simulink model "IndustrialMicrogrid"  (R2023a)
settings: Solver=FixedStepDiscrete  StartTime=0.0  StopTime=10  FixedStep=Ts  RelTol=1e-3
PostLoadFcn:
  | IndustrialMicrogridInputData
  | GfmGridFormingConverterInputParameters
model workspace (MAT data in the model file):
  caseNum = 2
undefined symbols (not defined in the file): base, BESS, DiscIntNeverNeededParam, grid, Grid, gridInverter, machine, microgrid, PV, PVInverter, PVTransformer, scrFactorRg, scrFactorXg, transformer, Ts
libraries: ee_lib x112, eeGeneralControl x104, nesl_utility_internal x64, simulink x56, nesl_utility x37, fl_lib x29, slpidlib x13, eeTransforms x11, eeTotalHarmonicDistorsion x8, eeRmsMeasurement x4, eeSinusoidalMeasurement x4, simulink_extras x2
(part 4 of 14)

== system IndustrialMicrogrid/MG2 Processing, Lighting and Auxiliary Loads/Motor Loads ==
  ASM measurement : ee_lib/Electromechanical/Asynchronous/Induction Machine Measurement  output_idx=11
      settings: InternalSimscapePortConfiguration="{\"Bottom\":[],\"Left\":[{\"id\":\"pu_input\",\"label\":\"pu\",\"type\":\"input\"}],\"Right\":[{\"id\":\"pu_output\",\"label\":\"o\",\"type\":\"output\"}],\"Top\":[]}"
  ASM measurement1 : ee_lib/Electromechanical/Asynchronous/Induction Machine Measurement  output_idx=12
      settings: InternalSimscapePortConfiguration="{\"Bottom\":[],\"Left\":[{\"id\":\"pu_input\",\"label\":\"pu\",\"type\":\"input\"}],\"Right\":[{\"id\":\"pu_output\",\"label\":\"o\",\"type\":\"output\"}],\"Top\":[]}"
  ASM measurement2 : ee_lib/Electromechanical/Asynchronous/Induction Machine Measurement  output_idx=12
      settings: InternalSimscapePortConfiguration="{\"Bottom\":[],\"Left\":[{\"id\":\"pu_input\",\"label\":\"pu\",\"type\":\"input\"}],\"Right\":[{\"id\":\"pu_output\",\"label\":\"o\",\"type\":\"output\"}],\"Top\":[]}"
  Asynchronous Machine Squirrel Cage (fundamental) : ee_lib/Electromechanical/Asynchronous/Induction Machine Squirrel Cage  port_option=ee.enum.threePhasePort.composite  SRated=750000 V*A  VRated=4160 V  FRated=60 Hz  nPolePairs=2  param_unit=ee.enum.unit.si  squirrel_cage=ee.enum.squirrelcage.Single  zero_sequence=ee.enum.park.zerosequence.exclude  initialization_option=ee.enum.asm.initialization.steadystate  Rs=0.016744*7 Ohm  Xls=0.035490*7 Ohm  pu_Rs=0.0258  pu_Lls=0.0413  Rrd=0.009857*7 Ohm  Xlrd=0.04280*7 Ohm  pu_Rrd=0.0145  pu_Llrd=0.0424  Rrd1=0.28 Ohm  Xlrd1=0.82 Ohm  Rrd2=0.28 Ohm  Xlrd2=0.82 Ohm  pu_Rrd1=0.0290  pu_Llrd1=0.0848  pu_Rrd2=0.0290  pu_Llrd2=0.0848  Xm=111.90*7 Ohm  pu_Lm=1.7562  X0=0.4*7 Ohm  pu_L0=0.0413  saturation_option=ee.enum.saturation.exclude  saturation_i=[0, 4, 9, 18, 25, 34, 50, 68, 95, 120] A  saturation_v=[0, 88, 154, 198, 220, 242, 264, 286, 308, 327] V  pu_saturation_i=[0, .176, .396, .792, 1.1, 1.496, 2.2, 2.992, 4.18, 5.28]  pu_saturation_v=[0, .4, .7, .9, 1, 1.1, 1.2, 1.3, 1.4, 1.4864]  connection_option=ee.enum.Connection.delta1  angular_position_specify=off  angular_position_priority=None  angular_position=0 deg  angular_position_nominal_specify=off  angular_position_nominal_unit=deg  angular_position_nominal_value=1  pu_psids_specify=off  pu_psids_priority=None  pu_psids=0  pu_psids_nominal_specify=off  pu_psids_nominal_unit=1  pu_psids_nominal_value=1  pu_psiqs_specify=off  pu_psiqs_priority=None  pu_psiqs=0  pu_psiqs_nominal_specify=off  pu_psiqs_nominal_unit=1  pu_psiqs_nominal_value=1  pu_psi0s_specify=off  pu_psi0s_priority=None  pu_psi0s=0  pu_psi0s_nominal_specify=off  pu_psi0s_nominal_unit=1  pu_psi0s_nominal_value=1  pu_psidr_specify=off  pu_psidr_priority=None  pu_psidr=0  pu_psidr_nominal_specify=off  pu_psidr_nominal_unit=1  pu_psidr_nominal_value=1  pu_psiqr_specify=off  pu_psiqr_priority=None  pu_psiqr=0  pu_psiqr_nominal_specify=off  pu_psiqr_nominal_unit=1  pu_psiqr_nominal_value=1  pu_psidr1_specify=off  pu_psidr1_priority=None  pu_psidr1=0  pu_psidr1_nominal_specify=off  pu_psidr1_nominal_unit=1  pu_psidr1_nominal_value=1  pu_psiqr1_specify=off  pu_psiqr1_priority=None  pu_psiqr1=0  pu_psiqr1_nominal_specify=off  pu_psiqr1_nominal_unit=1  pu_psiqr1_nominal_value=1  pu_psidr2_specify=off  pu_psidr2_priority=None  pu_psidr2=0  pu_psidr2_nominal_specify=off  pu_psidr2_nominal_unit=1  pu_psidr2_nominal_value=1  pu_psiqr2_specify=off  pu_psiqr2_priority=None  pu_psiqr2=0  pu_psiqr2_nominal_specify=off  pu_psiqr2_nominal_unit=1  pu_psiqr2_nominal_value=1  psids_specify=off  psids_priority=None  psids=0 Wb  psids_nominal_specify=off  psids_nominal_unit=Wb  psids_nominal_value=1  psiqs_specify=off  psiqs_priority=None  psiqs=0 Wb  psiqs_nominal_specify=off  psiqs_nominal_unit=Wb  psiqs_nominal_value=1  psi0s_specify=off  psi0s_priority=None  psi0s=0 Wb  psi0s_nominal_specify=off  psi0s_nominal_unit=Wb  psi0s_nominal_value=1  psidr_specify=off  psidr_priority=None  psidr=0 Wb  psidr_nominal_specify=off  psidr_nominal_unit=Wb  psidr_nominal_value=1  psiqr_specify=off  psiqr_priority=None  psiqr=0 Wb  psiqr_nominal_specify=off  psiqr_nominal_unit=Wb  psiqr_nominal_value=1  psidr1_specify=off  psidr1_priority=None  psidr1=0 Wb  psidr1_nominal_specify=off  psidr1_nominal_unit=Wb  psidr1_nominal_value=1  psiqr1_specify=off  psiqr1_priority=None  psiqr1=0 Wb  psiqr1_nominal_specify=off  psiqr1_nominal_unit=Wb  psiqr1_nominal_value=1  psidr2_specify=off  psidr2_priority=None  psidr2=0 Wb  psidr2_nominal_specify=off  psidr2_nominal_unit=Wb  psidr2_nominal_value=1  psiqr2_specify=off  psiqr2_priority=None  psiqr2=0 Wb  psiqr2_nominal_specify=off  psiqr2_nominal_unit=Wb  psiqr2_nominal_value=1  slip_specify=off  slip_priority=None  slip=0  slip_nominal_specify=off  slip_nominal_unit=1  slip_nominal_value=1  real_power_generated_specify=off  real_power_generated_priority=None  real_power_generated=0 W  real_power_generated_nominal_specify=off  real_power_generated_nominal_unit=W  real_power_generated_nominal_value=1  mechanical_power_consumed_specify=off  mechanical_power_consumed_priority=None  mechanical_power_consumed=0 W  mechanical_power_consumed_nominal_specify=off  mechanical_power_consumed_nominal_unit=W  mechanical_power_consumed_nominal_value=1  Tmeas=298.15 K  alpha=3.93e-3 1/K  alpha_cage=4.4e-3 1/K  stator_thermal_mass=100 J/K  rotor_thermal_mass=200 J/K  temperatureA_specify=off  temperatureA_priority=High  temperatureA=25 degC  temperatureA_nominal_specify=off  temperatureA_nominal_unit=degC  temperatureA_nominal_value=1  temperatureB_specify=off  temperatureB_priority=High  temperatureB=25 degC  temperatureB_nominal_specify=off  temperatureB_nominal_unit=degC  temperatureB_nominal_value=1  temperatureC_specify=off  temperatureC_priority=High  temperatureC=25 degC  temperatureC_nominal_specify=off  temperatureC_nominal_unit=degC  temperatureC_nominal_value=1  temperatureR_specify=off  temperatureR_priority=High  temperatureR=25 degC  temperatureR_nominal_specify=off  temperatureR_nominal_unit=degC  temperatureR_nominal_value=1
      settings: InternalSimscapePortConfiguration="{\"Bottom\":[],\"Left\":[{\"id\":\"R\",\"label\":\"R\",\"type\":\"foundation.mechanical.rotational.rotational\"},{\"id\":\"C\",\"label\":\"C\",\"type\":\"foundation.mechanical.rotational.rotational\"}],\"Right\":[{\"id\":\"pu_output\",\"label\":\"pu\",\"type\":\"output\"},{\"id\":\"N1\",\"label\":\"~1\",\"type\":\"foundation.electrical.three_phase\"},{\"id\":\"N2\",\"label\":\"~2\",\"type\":\"foundation.electrical.three_phase\"}],\"Top\":[]}"
  Electrical Reference1 : fl_lib/Electrical/Electrical Elements/Electrical Reference
  Generator : Scope  NumInputPorts=3
  Generator Sign Convention : Gain  Gain=-1
  Generator Sign Convention1 : Gain  Gain=-1
  Neutral Port (Three-Phase) : ee_lib/Connectors & References/Neutral Port (Three-Phase)  G_parasitic=1e-12 1/Ohm
      settings: InternalSimscapePortConfiguration="{\"Bottom\":[],\"Left\":[{\"id\":\"N\",\"label\":\"~\",\"type\":\"foundation.electrical.three_phase\"}],\"Right\":[{\"id\":\"n\",\"label\":\"n\",\"type\":\"foundation.electrical.electrical\"}],\"Top\":[]}"
  PS-Simulink Converter1 : nesl_utility/PS-Simulink Converter  PhysicalDomain=network_engine_domain  SubClassName=ps_output  LeftPortType=input  RightPortType=output  PseudoPeriodic=off  Frequencies=[]  VectorFormat=1-D array  Unit=1  AffineConversion=off
  PS-Simulink Converter2 : nesl_utility/PS-Simulink Converter  PhysicalDomain=network_engine_domain  SubClassName=ps_output  LeftPortType=input  RightPortType=output  PseudoPeriodic=off  Frequencies=[]  VectorFormat=1-D array  Unit=1  AffineConversion=off
  PS-Simulink Converter3 : nesl_utility/PS-Simulink Converter  PhysicalDomain=network_engine_domain  SubClassName=ps_output  LeftPortType=input  RightPortType=output  PseudoPeriodic=off  Frequencies=[]  VectorFormat=1-D array  Unit=1  AffineConversion=off
  Subsystem : Subsystem
  Two-Winding Transformer (Three-Phase)1 : ee_lib/Passive/Transformers/Two-Winding Transformer (Three-Phase)  SRated=microgrid.unitSubstationTransformerRating A*V  FRated=microgrid.frequency Hz  Winding1Connection=ee.enum.windingconnection.Y  VRated1=microgrid.powerCenterVoltage V  Winding2Connection=ee.enum.windingconnection.Y  VRated2=microgrid.powerCenterVoltage V  CoreType=ee.enum.coretype.threelimb  pu_Rw1=microgrid.unitSubstationPrimaryResistance  pu_Rw2=microgrid.unitSubstationPrimaryReactance*2  leakage_reactance_option=ee.enum.transformer_leakage.include  pu_Xl1=microgrid.unitSubstationSecondaryResistance  pu_Xl2=microgrid.unitSubstationSecondaryReactance*2  magnetizing_resistance_option=ee.enum.transformer_magnetizingResistance.include  pu_Rm=500  magnetizing_reactance_option=ee.enum.transformer_magnetizingReactance.include  saturation_option=ee.enum.transformer_saturation.exclude  pu_Xm=500  current_data=[0, .002, 1, 2]  magnetic_flux_data=[0, 1.2, 1.5, 1.51]  pu_X0=0.5  i1_specify=on  i1_priority=None  i1=[0, 0, 0] A  i1_nominal_specify=off  i1_nominal_unit=A  i1_nominal_value=1  i2_specify=on  i2_priority=None  i2=[0, 0, 0] A  i2_nominal_specify=off  i2_nominal_unit=A  i2_nominal_value=1  phi_specify=off  phi_priority=None  phi=[0, 0, 0]  phi_nominal_specify=off  phi_nominal_unit=1  phi_nominal_value=1  power_dissipated_specify=off  power_dissipated_priority=None  power_dissipated=0 W  power_dissipated_nominal_specify=off  power_dissipated_nominal_unit=W  power_dissipated_nominal_value=1
      settings: InternalSimscapePortConfiguration="{\"Bottom\":[],\"Left\":[{\"id\":\"N1\",\"label\":\"~1\",\"type\":\"foundation.electrical.three_phase\"}],\"Right\":[{\"id\":\"N2\",\"label\":\"~2\",\"type\":\"foundation.electrical.three_phase\"}],\"Top\":[]}"
  Conn2 : PMIOPort  Side=Right
  wires:
  PS-Simulink Converter1/1 -> Generator Sign Convention1/1
  Generator Sign Convention/1 -> Generator/1  "Real Power, pu"
  PS-Simulink Converter2/1 -> Generator Sign Convention/1
  Generator Sign Convention1/1 -> Generator/2  "Reactive Power, pu"
  PS-Simulink Converter3/1 -> Generator/3
  connections:
  ASM measurement/LConn1 -- ASM measurement1/LConn1 -- Asynchronous Machine Squirrel Cage (fundamental)/RConn1 -- ASM measurement2/LConn1
  Subsystem/LConn2 -- Asynchronous Machine Squirrel Cage (fundamental)/LConn2
  Subsystem/LConn1 -- Asynchronous Machine Squirrel Cage (fundamental)/LConn1
  Neutral Port (Three-Phase)/RConn1 -- Electrical Reference1/LConn1
  ASM measurement/RConn1 -- PS-Simulink Converter2/LConn1
  Two-Winding Transformer (Three-Phase)1/RConn1 -- Conn2/RConn1
  Asynchronous Machine Squirrel Cage (fundamental)/RConn3 -- Neutral Port (Three-Phase)/LConn1
  PS-Simulink Converter3/LConn1 -- ASM measurement2/RConn1
  ASM measurement1/RConn1 -- PS-Simulink Converter1/LConn1
  Asynchronous Machine Squirrel Cage (fundamental)/RConn2 -- Two-Winding Transformer (Three-Phase)1/LConn1

== system IndustrialMicrogrid/Operator Room/OperatorControlRoom ==
  mLoad : Inport
  mLoad2 : Inport  Port=2
  MGController2 : Inport  Port=3
  mPV : Inport  Port=4
  MGController1 : Inport  Port=5
  Tieline1 : Inport  Port=6
  mLoad3 : Inport  Port=7
  mDiesel : Inport  Port=8
  Tieline : Inport  Port=9
  "MG1 Controller : Commands and Measurements" : Subsystem
  "MG2 Controller : Commands and Measurements" : Subsystem
  Control Room MG1 : Outport
  Control Room MG2 : Outport  Port=2
  wires:
  mLoad/1 -> "MG1 Controller : Commands and Measurements"/1(mLoad)
  MGController1/1 -> "MG1 Controller : Commands and Measurements"/2(MGController1)
  "MG1 Controller : Commands and Measurements"/1(ControlRoom) -> Control Room MG1/1
  mLoad2/1 -> "MG2 Controller : Commands and Measurements"/1(mLoad2)
  MGController2/1 -> "MG2 Controller : Commands and Measurements"/2(MGController2)
  mPV/1 -> "MG2 Controller : Commands and Measurements"/3(mPV)
  mDiesel/1 -> "MG2 Controller : Commands and Measurements"/4(mDiesel)
  "MG2 Controller : Commands and Measurements"/1(ControlRoom) -> Control Room MG2/1
  Tieline1/1 -> "MG1 Controller : Commands and Measurements"/3(Tieline)
  Tieline/1 -> "MG2 Controller : Commands and Measurements"/5(mTieline)
  mLoad3/1 -> "MG1 Controller : Commands and Measurements"/4(mLoad3)

== system IndustrialMicrogrid/Operator Room/Signal Selector ==
  Control Room MG1 : Inport
  Control Room MG2 : Inport  Port=2
  "Control Room MG1 " : InportShadow
  Control Room MG1 1 : InportShadow
  Control Room MG1 2 : InportShadow
  "Control Room MG2 " : InportShadow  Port=2
  Control Room MG2 1 : InportShadow  Port=2
  MG1 Load : Subsystem
  MG1 Portable Substation : Subsystem
  MG1 Primary Substation : Subsystem
  MG1 Unit Substation : Subsystem
  MG2 Load : Subsystem
  MG2 Power Center : Subsystem
  MG2 Primary Substation : Subsystem
  Primary Substation 1 : Outport
  Primary Substation 2 : Outport  Port=2
  Unit Substation : Outport  Port=3
  Power Center : Outport  Port=4
  Drilling Load : Outport  Port=5
  "Processing, and Auxiliary Loads " : Outport  Port=6
  Portable Substation : Outport  Port=7
  wires:
  Control Room MG1/1 -> MG1 Primary Substation/1(In1)
  MG1 Primary Substation/1(Primary Substation 1) -> Primary Substation 1/1
  Control Room MG2/1 -> MG2 Primary Substation/1(In1)
  MG2 Primary Substation/1(Primary Substation 2) -> Primary Substation 2/1
  "Control Room MG1 "/1 -> MG1 Unit Substation/1(In1)
  MG1 Unit Substation/1(Out1) -> Unit Substation/1
  "Control Room MG2 "/1 -> MG2 Power Center/1(In1)
  MG2 Power Center/1(Out1) -> Power Center/1
  Control Room MG1 1/1 -> MG1 Load/1(In1)
  MG1 Load/1(Out1) -> Drilling Load/1
  Control Room MG2 1/1 -> MG2 Load/1(In1)
  MG2 Load/1(Out1) -> "Processing, and Auxiliary Loads "/1
  Control Room MG1 2/1 -> MG1 Portable Substation/1(In1)
  MG1 Portable Substation/1(Portable Substation) -> Portable Substation/1

== system IndustrialMicrogrid/Selected Results/MG1 ==
  In Bus Element29 : Inport  PortName=MGController1  Element=BESS.active power
  In Bus Element30 : Inport  PortName=MGController1  Element=BESS.reactive power
  In Bus Element1 : Inport  PortName=MGController1  Element=BESS.voltage
  In Bus Element3 : Inport  PortName=MGController1  Element=BESS.voltage
  In Bus Element2 : Inport  PortName=MGController1  Element=BESS.current
  In Bus Element4 : Inport  PortName=MGController1  Element=BESS.current
  In Bus Element27 : Inport  PortName=MGController1  Element=Controller.ResynchMGController.PCC measurments.PCC.mPCC.activepower
  In Bus Element28 : Inport  PortName=MGController1  Element=Controller.ResynchMGController.PCC measurments.PCC.mPCC.reactivepower
  In Bus Element25 : Inport  Port=2  PortName=mLoad  Element=active power
  In Bus Element26 : Inport  Port=2  PortName=mLoad  Element=reactive power
  BESS Measurements : Scope  NumInputPorts=4
  Bus Creator : BusCreator  Inputs=3
  Bus Creator1 : BusCreator  Inputs=3
  Gain : Gain
  Gain1 : Gain
  "Inverter Active & Reactive Power " : Subsystem
  Power  Measurements : Scope  NumInputPorts=2
  Terminator : Terminator
  Terminator1 : Terminator
  wires:
  In Bus Element29/1 -> Bus Creator/2  "BESS Active Power"
  Bus Creator/1 -> Power  Measurements/1
  In Bus Element30/1 -> Bus Creator1/2  "BESS Reactive Power"
  Bus Creator1/1 -> Power  Measurements/2
  In Bus Element25/1 -> Bus Creator/3  "Load Active Power"
  In Bus Element27/1 -> Bus Creator/1  "Grid Active Power"
  In Bus Element28/1 -> Bus Creator1/1  "Grid Reactive Power"
  In Bus Element26/1 -> Bus Creator1/3  "Load Reactive Power"
  In Bus Element4/1 -> BESS Measurements/4  "BESS Current (pu)"
  "Inverter Active & Reactive Power "/2(Q) -> Gain1/1, BESS Measurements/2  "BESS  Reactive Power (pu)"
  In Bus Element2/1 -> "Inverter Active & Reactive Power "/2(Iabc)  "BESS Current (pu)"
  In Bus Element3/1 -> BESS Measurements/3  "BESS Voltage (pu)"
  "Inverter Active & Reactive Power "/1(P) -> Gain/1, BESS Measurements/1  "BESS  Active Power (pu)"
  In Bus Element1/1 -> "Inverter Active & Reactive Power "/1(Vabc)  "BESS Voltage (pu)"
  Gain/1 -> Terminator/1  "P BESS MG1"
  Gain1/1 -> Terminator1/1  "Q BESS MG1"

== system IndustrialMicrogrid/Selected Results/MG2 ==
  In Bus Element12 : Inport  PortName=MGController2  Element=BESS2.active power
  In Bus Element13 : Inport  PortName=MGController2  Element=BESS2.reactive power
  In Bus Element5 : Inport  PortName=MGController2  Element=BESS2.voltage
  In Bus Element7 : Inport  PortName=MGController2  Element=BESS2.voltage
  In Bus Element6 : Inport  PortName=MGController2  Element=BESS2.current
  In Bus Element8 : Inport  PortName=MGController2  Element=BESS2.current
  In Bus Element10 : Inport  PortName=MGController2  Element=MGController2.IslandMGController2.PCC measurments2.PCC2.mPCC2.activepower
  In Bus Element11 : Inport  PortName=MGController2  Element=MGController2.ResynchMGController2.PCC measurments2.PCC2.mPCC2.reactivepower
  In Bus Element14 : Inport  Port=2  PortName=mLoad2  Element=active power
  In Bus Element15 : Inport  Port=2  PortName=mLoad2  Element=reactive power
  In Bus Element17 : Inport  Port=3  PortName=mPV  Element=mPV.ActivePower
  In Bus Element18 : Inport  Port=3  PortName=mPV  Element=mPV.RectivePower
  In Bus Element19 : Inport  Port=4  PortName=mdiesel  Element=active power
  In Bus Element20 : Inport  Port=4  PortName=mdiesel  Element=reactive power
  BESS Measurements1 : Scope  NumInputPorts=4
  Bus Creator2 : BusCreator  Commented=on  Inputs=5
  Bus Creator3 : BusCreator  Commented=on  Inputs=5
  Bus Creator4 : BusCreator  Inputs=5
  Bus Creator5 : BusCreator  Inputs=5
  Gain : Gain
  Gain1 : Gain
  Inverter Active & Reactive Power 1 : Subsystem
  Power  Measurements1 : Scope  NumInputPorts=2
  Terminator : Terminator
  Terminator1 : Terminator
  wires:
  In Bus Element8/1 -> BESS Measurements1/4  "BESS Current (pu)"
  In Bus Element7/1 -> BESS Measurements1/3  "BESS Voltage (pu)"
  In Bus Element6/1 -> Inverter Active & Reactive Power 1/2(Iabc)  "BESS Active Power"
  In Bus Element5/1 -> Inverter Active & Reactive Power 1/1(Vabc)  "BESS Active Power"
  Bus Creator5/1 -> Power  Measurements1/2
  In Bus Element15/1 -> Bus Creator5/3  "Load Reactive Power"
  In Bus Element12/1 -> Bus Creator4/2  "BESS Active Power"
  In Bus Element17/1 -> Bus Creator4/4  "PV Active Power"
  In Bus Element10/1 -> Bus Creator4/1  "Grid Active Power"
  In Bus Element20/1 -> Bus Creator5/5  "Diesel Reactive Power"
  In Bus Element13/1 -> Bus Creator5/2  "BESS Reactive Power"
  In Bus Element11/1 -> Bus Creator5/1  "Grid Reactive Power"
  In Bus Element19/1 -> Bus Creator4/5  "Diesl Active Power"
  In Bus Element18/1 -> Bus Creator5/4  "PV Rective Power"
  In Bus Element14/1 -> Bus Creator4/3  "Load Active Power"
  Bus Creator4/1 -> Power  Measurements1/1
  Gain1/1 -> Terminator1/1  "Q BESS MG2"
  Gain/1 -> Terminator/1  "P BESS MG2"
  Inverter Active & Reactive Power 1/1(P) -> Gain/1, BESS Measurements1/1  "BESS  Active Power (pu)"
  Inverter Active & Reactive Power 1/2(Q) -> Gain1/1, BESS Measurements1/2  "BESS  Reactive Power (pu)"

== system IndustrialMicrogrid/MG1 Drilling Loads/Subsystem2/Subsystem ==
  Gain : Gain  Gain=60/(2*pi)
  Ideal Rotational Motion Sensor : fl_lib/Mechanical/Mechanical Sensors/Ideal Rotational Motion Sensor  reference=foundation.enum.MeasurementReference.difference  acceleration_port=false  velocity_port=true  position_port=false  wrap_angle=false  offset=0 rad
      settings: InternalSimscapePortConfiguration="{\"Bottom\":[],\"Left\":[{\"id\":\"R\",\"label\":\"R\",\"type\":\"foundation.mechanical.rotational.rotational\"}],\"Right\":[{\"id\":\"C\",\"label\":\"C\",\"type\":\"foundation.mechanical.rotational.rotational\"},{\"id\":\"W\",\"label\":\"W\",\"type\":\"output\"}],\"Top\":[]}"
  Machine Mechanical Power : ee_lib/Electromechanical/Mechanical/Machine Mechanical Power  power_sign=1  SRated=132000 A*V  FRated=60 Hz  nPolePairs=2  inputUnit=ee.enum.unit.si  torque_factor=2  inertia_option=2  J=10 kg*m^2  H=3.525 W*s/(A*V)  damper_option=2  D=39.0509 N*m*s/rad  pu_D=0.01  initialization_option=2  fMechanical0=60 Hz  fElectrical0=60 Hz
      settings: InternalSimscapePortConfiguration="{\"Bottom\":[],\"Left\":[{\"id\":\"Pm\",\"label\":\"Pm\",\"type\":\"input\"}],\"Right\":[{\"id\":\"R\",\"label\":\"R\",\"type\":\"foundation.mechanical.rotational.rotational\"},{\"id\":\"C\",\"label\":\"C\",\"type\":\"foundation.mechanical.rotational.rotational\"}],\"Top\":[]}"
  Mechanical Rotational Reference : fl_lib/Mechanical/Rotational Elements/Mechanical Rotational Reference
  PS-Simulink Converter : nesl_utility/PS-Simulink Converter  PhysicalDomain=network_engine_domain  SubClassName=ps_output  LeftPortType=input  RightPortType=output  PseudoPeriodic=off  Frequencies=[]  VectorFormat=inherit  Unit=inherit  AffineConversion=off
  Power : Constant  Value=120000
  Scope : Scope
  Simulink-PS Converter2 : nesl_utility/Simulink-PS Converter  PhysicalDomain=network_engine_domain  SubClassName=ps_input  LeftPortType=input  RightPortType=output  PseudoPeriodic=off  Frequencies=[]  NoiseDistribution=none  NoiseParameters=[]  Unit=1  AffineConversion=off  FilteringAndDerivatives=provide  SimscapeFilterOrder=1  InputFilterTimeConstant=0.001  UdotUserProvided=0
  Conn1 : PMIOPort  Side=Left
  Conn2 : PMIOPort  Port=2  Side=Left
  wires:
  PS-Simulink Converter/1 -> Gain/1
  Gain/1 -> Scope/1
  Power/1 -> Simulink-PS Converter2/1
  connections:
  PS-Simulink Converter/LConn1 -- Ideal Rotational Motion Sensor/RConn2
  Simulink-PS Converter2/RConn1 -- Machine Mechanical Power/LConn1
  Conn1/RConn1 -- Ideal Rotational Motion Sensor/LConn1 -- Machine Mechanical Power/RConn1
  Conn2/RConn1 -- Mechanical Rotational Reference/LConn1 -- Machine Mechanical Power/RConn2 -- Ideal Rotational Motion Sensor/RConn1

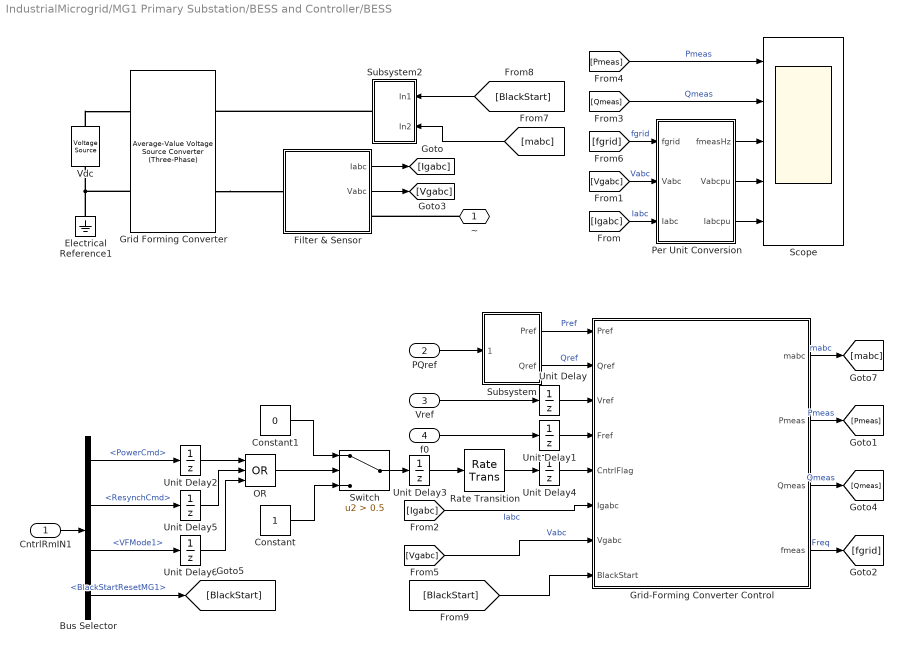
== system IndustrialMicrogrid/MG1 Primary Substation/BESS and Controller/BESS ==
  CntrlRmIN1 : Inport
  PQref : Inport  Port=2
  Vref : Inport  Port=3
  f0 : Inport  Port=4
  Bus Selector : BusSelector  OutputSignals=PowerCmd,ResynchCmd,VFMode1,BlackStartResetMG1
  Constant : Constant
  Constant1 : Constant  Value=0
  Electrical Reference1 : fl_lib/Electrical/Electrical Elements/Electrical Reference
  Filter & Sensor : Subsystem
      mask Display: image('$imagefile'); % Use "Edit Image" on toolstrip to change.
  Grid Forming Converter : ee_lib/Semiconductors & Converters/Converters/Average-Value Voltage Source Converter (Three-Phase)  port_option=ee.enum.threePhasePort.composite  frequency_option=ee.enum.converters.frequency.variable  FRated=50 Hz  losses_parameterization=ee.enum.converters.losses.fixed  Pfixed=1 W  ks=0.01  kc1=1.7 V  kc2=0.01 Ohm  Ploss_vect=[100, 800, 1870, 3250, 4900] W  Irms_vect=[10, 100, 200, 300, 400] A  Vdc_nom=300 V  thermal_mass=30000 J/K  temperature_specify=off  temperature_priority=High  temperature=298.15 K  temperature_nominal_specify=off  temperature_nominal_unit=K  temperature_nominal_value=1
      settings: InternalSimscapePortConfiguration="{\"Bottom\":[],\"Left\":[{\"id\":\"ModWave\",\"label\":\"ModWave\",\"type\":\"input\"},{\"id\":\"N\",\"label\":\"~\",\"type\":\"foundation.electrical.three_phase\"}],\"Right\":[{\"id\":\"p\",\"label\":\"+\",\"type\":\"foundation.electrical.electrical\"},{\"id\":\"n\",\"label\":\"-\",\"type\":\"foundation.electrical.electrical\"}],\"Top\":[]}"
  Grid-Forming Converter Control : Subsystem  mask(Grid Forming Controller){power=gridInverter.apparentPower*1e3, girdLineVoltage=gridInverter.lineRMSVoltage, powerFreq=gridInverter.frequency, dcBusVoltage=gridInverter.DCVoltage, measSampleTime=gridInverter.measurementSampleTime, powerControl=Virtual Synchronous Machine, activePowerSampleTime=gridInverter.droopControl.sampleTime, droopSlope=gridInverter.droopControl.freqSlopeMp, droopT1=gridInverter.droopControl.T1, droopT2=gridInverter.droopControl.T2, droopTC=gridInverter.droopControl.lpfTimeConst, vsmPmeasFilterTC=gridInverter.vsm.PmeasTimeConst, vsmFreqDroop=gridInverter.vsm.freqDroop, vsmInertiaTC=gridInverter.vsm.inertiaConstant, vsmDampingConst=gridInverter.vsm.dampingCoefficent, dampingPowerMaxLimit=gridInverter.vsm.maxDampingPower, dampingPowerMinLimit=gridInverter.vsm.minDampingPower, freqMeasTimeConst=gridInverter.freqMeasTimeConst, freqOption=Constant Frequency Reference, voltreference=gridInverter.Qcontrol.voltageReference, QVoltFilterTC=gridInverter.Qcontrol.QmeasTimeConst, QVoltDroop=gridInverter.Qcontrol.voltageDroop, currentLimit=Virtual Impedance, maxSatCurrentLimit=gridInverter.currentLimit.maxSaturationCurrent, maxVICurrentLimit=gridInverter.currentLimit.viCurrentLimit, ctLimitVirtualImp=gridInverter.currentLimit.virImpResistanceCoeff, ctLimitXbyR=gridInverter.currentLimit.virImpXbyR, ctLimitDelayTime=gridInverter.currentLimit.maxSaturationDelay, currentSatTime=gridInverter.currentLimit.satCurrentRunTime, currentVITimeConst=gridInverter.currentLimit.viFilterTimeConst, voltControlTs=gridInverter.controller.VoltageControlSampleTime, vdPGain=gridInverter.controller.voltControllerKp, VdIGain=gridInverter.controller.voltControllerKi, VdMaxCt=gridInverter.controller.voltageMaxId, VdMinCt=gridInverter.controller.voltageMinId, VqPGain=gridInverter.controller.voltControllerKp, VqIGain=gridInverter.controller.voltControllerKi, VqMaxCt=gridInverter.controller.voltageMaxIq, VqMinCt=gridInverter.controller.voltageMinIq, vdvqLPFTimeConst=gridInverter.controller.voltMeasTimeConst, currentControlTs=gridInverter.controller.CurrentControlSampleTime, filterInductance=gridInverter.L, IdPGain=gridInverter.controller.ctControllerKp, IdIGain=gridInverter.controller.ctControllerKi, IqPGain=gridInverter.controller.ctControllerKp, IqIGain=gridInverter.controller.ctControllerKi}
      mask prompts: power "Grid forming converter power (VA)"; girdLineVoltage "Grid line voltage (V)"; powerFreq "Grid frequency (Hz)"; dcBusVoltage "DC bus voltage"; measSampleTime "Measurement sample time"; powerControl "Active Power Control"; activePowerSampleTime "Sample time (s)"; droopSlope "Power droop slope (pu, Hz/W)"; droopT1 "Lead-Lag numerator time constant (s)"; droopT2 "Lead-Lag denominator time constant (s)"; droopTC "Filter cut-off time constant (s)"; vsmPmeasFilterTC "Power measurement filter time constant (s)"; vsmFreqDroop "Frequency droop (pu,  W/Hz)"; vsmInertiaTC "Inertia constant M (pu)"; vsmDampingConst "Damping constant (pu/Hz)"; dampingPowerMaxLimit "Damping power maximum limit (pu)"; dampingPowerMinLimit "Damping power minimum limit (pu)"; freqMeasTimeConst "Frequency measurement time constant (s)"; freqOption "Damping power fequency option"; voltreference "Voltage reference value (pu)"; QVoltFilterTC "Power measurement filter time constant (s)"; QVoltDroop "Voltage droop (pu, V/VAR)"; currentLimit "Current limiting method"; maxSatCurrentLimit "Maximum current saturation (pu)"; maxVICurrentLimit "Maximum virtual impedance current (pu)"; ctLimitVirtualImp "Virtual impedance coefficient (pu.Ohm/pu.A)"; ctLimitXbyR "Virtual X/R ratio"; ctLimitDelayTime "Maximum current delay time (s)"; currentSatTime "Current limiting run time (s)"; currentVITimeConst "Filter time constant (s)"; voltControlTs "Controller sample time (s)"; vdPGain "Vd proportional gain"; VdIGain "Vd integral gain"; VdMaxCt "Vd maximum current limit (A)"; VdMinCt "Vd minimum current limit (A)"; VqPGain "Vq proportional gain"; VqIGain "Vq integral gain"; VqMaxCt "Vq maximum current limit (A)"; VqMinCt "Vq minimum current limit (A)"; vdvqLPFTimeConst "Voltage measurement filter time constant (s)"; currentControlTs "Controller sample time (s)"; filterInductance "Filter inductance (H)"; IdPGain "Id proportional gain"; IdIGain "Id integral gain"; IqPGain "Iq proportional gain"; IqIGain "Iq integral gain"
      mask help: This block implements the grid forming controller with fault ride through capability. Input to the controller are active and reactive power reference in per unit and the sensed three-phase phase current in amphere and phase voltage in volts.
      mask init:
      | powerChoice = get_param(gcb,'powerControl');
      | currentChoice = get_param(gcb,'currentLimit');
      | 
      | powerloc = [gcb, '/Power Control/ActivePowerControl']; 
      | currentloc = [gcb, '/Current Limiting/CurrentLimitingMethod'];
      | freqLoc = [gcb,'/Power Control/ActivePowerControl/vsmControl/Damping Frequency'];
      | 
      | switch powerChoice
      |     case 'Virtual Synchronous Machine'
      |         set_param(powerloc, 'LabelModeActiveChoice', 'vsm');
      |         dampingFreqChoice = get_param(gcb,'freqOption');
      |         if strcmp(dampingFreqChoice,'Use Grid Frequency Measurement')
      |             set_param(freqLoc, 'LabelModeActiveChoice', 'freqMeas');
      |         else
      |             set_param(freqLoc, 'LabelModeActiveChoice', 'constFreq');
      |         end
      |     case 'Droop Control'
      |          set_param(powerloc, 'LabelModeActiveChoice', 'droop');
      |    otherwise
      |         disp('Choose proper active power control method')
      | end
      | switch currentChoice
      |     case 'Virtual Impedance'
      |           set_param(currentloc, 'LabelModeActiveChoice', 'virimp');
      |     case 'Current Limiting'
      |          set_param(currentloc, 'LabelModeActiveChoice', 'ctSat');
      |     case 'Combining Virtual Impedance and Current Limiting'
      |             set_param(currentloc, 'LabelModeActiveChoice', 'both');
      |     otherwise
      |         disp('Choose proper current limiting method')
      | end
      mask TypeOptions powerControl: Virtual Synchronous Machine | Droop Control
      mask Callback powerControl:
      | h = Simulink.Mask.get(gcb);
      | slectedActivePowerControl=get_param(gcb,'powerControl');
      | %slectedActivePowerControl = h.Parameters(find(string({h.Parameters.Name}) == 'powerControl')).Value;
      | switch slectedActivePowerControl
      |     case 'Virtual Synchronous Machine'
      |         h.Parameters(find(string({h.Parameters.Name}) == 'droopSlope')).Visible = 'off';
      |         h.Parameters(find(string({h.Parameters.Name}) == 'droopTC')).Visible = 'off';
      |         h.Parameters(find(string({h.Parameters.Name}) == 'droopT1')).Visible = 'off';
      |         h.Parameters(find(string({h.Parameters.Name}) == 'droopT2')).Visible = 'off';
      |         h.Parameters(find(string({h.Parameters.Name}) == 'vsmPmeasFilterTC')).Visible = 'on';
      |         h.Parameters(find(string({h.Parameters.Name}) == 'vsmFreqDroop')).Visible = 'on';
      |         h.Parameters(find(string({h.Parameters.Name}) == 'vsmInertiaTC')).Visible = 'on';
      |         h.Parameters(find(string({h.Parameters.Name}) == 'vsmDampingConst')).Visible = 'on';
      |         h.Parameters(find(string({h.Parameters.Name}) == 'dampingPowerMaxLimit')).Visible = 'on';
      |         h.Parameters(find(string({h.Parameters.Name}) == 'dampingPowerMinLimit')).Visible = 'on';
      |         h.Parameters(find(string({h.Parameters.Name}) == 'freqOption')).Visible = 'on';
      |         h.Parameters(find(string({h.Parameters.Name}) == 'freqMeasTimeConst')).Visible = 'on';
      |     case 'Droop Control'
      |         h.Parameters(find(string({h.Parameters.Name}) == 'droopSlope')).Visible = 'on';
      |         h.Parameters(find(string({h.Parameters.Name}) == 'droopTC')).Visible = 'on';
      |         h.Parameters(find(string({h.Parameters.Name}) == 'droopT1')).Visible = 'on';
      |         h.Parameters(find(string({h.Parameters.Name}) == 'droopT2')).Visible = 'on';
      |         h.Parameters(find(string({h.Parameters.Name}) == 'vsmPmeasFilterTC')).Visible = 'off';
      |         h.Parameters(find(string({h.Parameters.Name}) == 'vsmFreqDroop')).Visible = 'off';
      |         h.Parameters(find(string({h.Parameters.Name}) == 'vsmInertiaTC')).Visible = 'off';
      |         h.Parameters(find(string({h.Parameters.Name}) == 'vsmDampingConst')).Visible = 'off';
      |         h.Parameters(find(string({h.Parameters.Name}) == 'dampingPowerMaxLimit')).Visible = 'off';
      |         h.Parameters(find(string({h.Parameters.Name}) == 'dampingPowerMinLimit')).Visible = 'off';
      |         h.Parameters(find(string({h.Parameters.Name}) == 'freqOption')).Visible = 'off';
      |         h.Parameters(find(string({h.Parameters.Name}) == 'freqMeasTimeConst')).Visible = 'on';
      | 
      |     otherwise
      |         disp('Choose proper active power control method')
      | end
      mask TypeOptions freqOption: Use Grid Frequency Measurement | Constant Frequency Reference
      mask TypeOptions currentLimit: Virtual Impedance | Current Limiting | Combining Virtual Impedance and Current Limiting
      mask Callback currentLimit:
      | currentLimit = 1;
      | h = Simulink.Mask.get(gcb);
      | currentLimitControl=get_param(gcb,'currentLimit');
      | %slectedActivePowerControl = h.Parameters(find(string({h.Parameters.Name}) == 'powerControl')).Value;
      | switch currentLimitControl
      |     case 'Virtual Impedance'
      |         h.Parameters(find(string({h.Parameters.Name}) == 'maxVICurrentLimit')).Visible = 'on';
      |         h.Parameters(find(string({h.Parameters.Name}) == 'ctLimitVirtualImp')).Visible = 'on';
      |         h.Parameters(find(string({h.Parameters.Name}) == 'ctLimitXbyR')).Visible = 'on';
      |         h.Parameters(find(string({h.Parameters.Name}) == 'maxSatCurrentLimit')).Visible = 'off';
      |         h.Parameters(find(string({h.Parameters.Name}) == 'ctLimitDelayTime')).Visible = 'off';
      |         h.Parameters(find(string({h.Parameters.Name}) == 'currentSatTime')).Visible = 'off';
      |         h.Parameters(find(string({h.Parameters.Name}) == 'currentVITimeConst')).Visible = 'on';
      | 
      | 
      |     case 'Current Limiting'
      |         h.Parameters(find(string({h.Parameters.Name}) == 'maxVICurrentLimit')).Visible = 'off';
      |         h.Parameters(find(string({h.Parameters.Name}) == 'ctLimitVirtualImp')).Visible = 'off';
      |         h.Parameters(find(string({h.Parameters.Name}) == 'ctLimitXbyR')).Visible = 'off';
      |         h.Parameters(find(string({h.Parameters.Name}) == 'maxSatCurrentLimit')).Visible = 'on';
      |         h.Parameters(find(string({h.Parameters.Name}) == 'ctLimitDelayTime')).Visible = 'on';
      |         h.Parameters(find(string({h.Parameters.Name}) == 'currentSatTime')).Visible = 'off';
      |         h.Parameters(find(string({h.Parameters.Name}) == 'currentVITimeConst')).Visible = 'off';
      | 
      |     case 'Combining Virtual Impedance and Current Limiting'
      |         h.Parameters(find(string({h.Parameters.Name}) == 'maxVICurrentLimit')).Visible = 'on';
      |         h.Parameters(find(string({h.Parameters.Name}) == 'ctLimitVirtualImp')).Visible = 'on';
      |         h.Parameters(find(string({h.Parameters.Name}) == 'ctLimitXbyR')).Visible = 'on';
      |         h.Parameters(find(string({h.Parameters.Name}) == 'maxSatCurrentLimit')).Visible = 'on';
      |         h.Parameters(find(string({h.Parameters.Name}) == 'ctLimitDelayTime')).Visible = 'off';
      |         h.Parameters(find(string({h.Parameters.Name}) == 'currentSatTime')).Visible = 'on';
      |         h.Parameters(find(string({h.Parameters.Name}) == 'currentVITimeConst')).Visible = 'on';
      | 
      |     otherwise
      |         disp('Choose proper current limiting method')
      | end
      mask DialogControl ParameterGroupVar Prompt: Grid Forming Control Parameters
      mask DialogControl Container8 Prompt: Grid-forming Converter Specification
      mask DialogControl Pcontrolgrp Prompt: Active Power Controller Parameters
      mask DialogControl QcontrolGrp Prompt: Reactive Power Controller Parameters
      mask DialogControl faultRideThroughGrp Prompt: Fault Ride Through Parameters
      mask DialogControl voltControlgrp Prompt: Voltage Controller Parameters
      mask DialogControl Container15currentContGrp Prompt: Current Controller Parameters
      mask Display: image('$imagefile'); % Use "Edit Image" on toolstrip to change.
  OR : Logic  Operator=OR  Inputs=3  IconShape=distinctive  AllPortsSameDT=off  OutDataTypeStr=boolean
  Per Unit Conversion : Subsystem
  Rate Transition : RateTransition
  Scope : Scope  NumInputPorts=5
  Subsystem : Subsystem
  Subsystem2 : Subsystem
  Switch : Switch  Criteria=u2 > Threshold  Threshold=0.5  SaturateOnIntegerOverflow=off  InputSameDT=off
  Unit Delay : UnitDelay  SampleTime=-1  HasFrameUpgradeWarning=on
  Unit Delay1 : UnitDelay  SampleTime=-1  HasFrameUpgradeWarning=on
  Unit Delay2 : UnitDelay  SampleTime=Ts  HasFrameUpgradeWarning=on
  Unit Delay3 : UnitDelay  InitialCondition=1  SampleTime=Ts  HasFrameUpgradeWarning=on
  Unit Delay4 : UnitDelay  InitialCondition=1  SampleTime=Ts  HasFrameUpgradeWarning=on
  Unit Delay5 : UnitDelay  SampleTime=Ts  HasFrameUpgradeWarning=on
  Unit Delay6 : UnitDelay  SampleTime=Ts  HasFrameUpgradeWarning=on
  Vdc : ee_lib/Sources/Voltage Source  dc_voltage=gridInverter.DCVoltage V  ac_voltage=0 V  ac_shift=0 rad  ac_frequency=0 Hz  noise_mode=ee.enum.sources.noise.Disabled  PSD=0 V^2/Hz  sample_time=1e-3 s  repeatability=ee.enum.sources.repeatability.NotRepeatable  user_seed=0  auto_seed=2016017452  i_specify=off  i_priority=None  i=0 A  i_nominal_specify=off  i_nominal_unit=A  i_nominal_value=1  v_specify=off  v_priority=None  v=0 V  v_nominal_specify=off  v_nominal_unit=V  v_nominal_value=1
  "~ " : PMIOPort  Side=Left
  wires:
  Grid-Forming Converter Control/3(Qmeas) -> [Qmeas]  "Qmeas"
  Grid-Forming Converter Control/2(Pmeas) -> [Pmeas]  "Pmeas"
  Filter & Sensor/2(Vabc) -> [Vgabc]
  Filter & Sensor/1(Iabc) -> [Igabc]
  [Vgabc] -> Grid-Forming Converter Control/7(Vgabc)  "Vabc"
  Subsystem/1(Pref) -> Grid-Forming Converter Control/1(Pref)  "Pref"
  Grid-Forming Converter Control/1(mabc) -> [mabc]  "mabc"
  Grid-Forming Converter Control/4(fmeas) -> [fgrid]  "Freq"
  Subsystem/2(Qref) -> Grid-Forming Converter Control/2(Qref)  "Qref"
  [Igabc] -> Grid-Forming Converter Control/6(Igabc)  "Iabc"
  Per Unit Conversion/3(Iabcpu) -> Scope/5
  Per Unit Conversion/2(Vabcpu) -> Scope/4
  Per Unit Conversion/1(fmeasHz) -> Scope/3
  [Pmeas] -> Scope/1  "Pmeas"
  [Qmeas] -> Scope/2  "Qmeas"
  [Igabc] -> Per Unit Conversion/3(Iabc)  "Iabc"
  [fgrid] -> Per Unit Conversion/1(fgrid)  "fgrid"
  [Vgabc] -> Per Unit Conversion/2(Vabc)  "Vabc"
  Bus Selector/1 -> Unit Delay2/1  "<PowerCmd>"
  CntrlRmIN1/1 -> Bus Selector/1
  f0/1 -> Unit Delay1/1
  Vref/1 -> Unit Delay/1
  PQref/1 -> Subsystem/1(PQref)
  Unit Delay/1 -> Grid-Forming Converter Control/3(Vref)
  Unit Delay1/1 -> Grid-Forming Converter Control/4(Fref)
  Switch/1 -> Unit Delay3/1
  Unit Delay3/1 -> Rate Transition/1
  Rate Transition/1 -> Unit Delay4/1
  Unit Delay4/1 -> Grid-Forming Converter Control/5(CntrlFlag)
  Constant/1 -> Switch/3
  Constant1/1 -> Switch/1
  Bus Selector/2 -> Unit Delay5/1  "<ResynchCmd>"
  Unit Delay2/1 -> OR/1
  Unit Delay5/1 -> OR/2
  OR/1 -> Switch/2
  Bus Selector/3 -> Unit Delay6/1  "<VFMode1>"
  Unit Delay6/1 -> OR/3
  [mabc] -> Subsystem2/2(In2)
  [BlackStart] -> Subsystem2/1(In1)
  Bus Selector/4 -> [BlackStart]  "<BlackStartResetMG1>"
  [BlackStart] -> Grid-Forming Converter Control/8(BlackStart)
  connections:
  Grid Forming Converter/RConn2 -- Vdc/RConn1 -- Electrical Reference1/LConn1
  "~ "/RConn1 -- Filter & Sensor/RConn1
  Grid Forming Converter/LConn2 -- Filter & Sensor/LConn1
  Vdc/LConn1 -- Grid Forming Converter/RConn1
  Subsystem2/RConn1 -- Grid Forming Converter/LConn1

== system IndustrialMicrogrid/MG1 Primary Substation/BESS and Controller/BESS Converter Measurement  ==
  Current and Voltage Sensor (Three-Phase) : ee_lib/Sensors & Transducers/Current and Voltage Sensor (Three-Phase)  vMeasurementType=ee.enum.vmeasurement.lg  outputUnit=ee.enum.unit.pu  SRated=1e6 A*V  VRated=microgrid.voltage V  I_specify=off  I_priority=None  I=[ 0 0 0 ] A  I_nominal_specify=off  I_nominal_unit=A  I_nominal_value=1  V_specify=off  V_priority=None  V=[ 0 0 0 ] V  V_nominal_specify=off  V_nominal_unit=V  V_nominal_value=1
      settings: InternalSimscapePortConfiguration="{\"Bottom\":[],\"Left\":[{\"id\":\"N1\",\"label\":\"~1\",\"type\":\"foundation.electrical.three_phase\"}],\"Right\":[{\"id\":\"V_output\",\"label\":\"V\",\"type\":\"output\"},{\"id\":\"I_output\",\"label\":\"I\",\"type\":\"output\"},{\"id\":\"N2\",\"label\":\"~2\",\"type\":\"foundation.electrical.three_phase\"}],\"Top\":[]}"
  Low-Pass Filter (Discrete or Continuous) : eeGeneralControl/Low-Pass Filter (Discrete or Continuous)  K=1  T=0.02  B=inf  A=-inf  init_option=Inherited from block input  x0=0  Ts=Ts
  Low-Pass Filter (Discrete or Continuous)1 : eeGeneralControl/Low-Pass Filter (Discrete or Continuous)  K=1  T=0.02  B=inf  A=-inf  init_option=Inherited from block input  x0=0  Ts=Ts
  PS-Simulink Converter2 : nesl_utility_internal/PS-Simulink Converter  PhysicalDomain=network_engine_domain  SubClassName=ps_output  LeftPortType=input  RightPortType=output  PseudoPeriodic=off  Frequencies=[]  VectorFormat=1-D array  Unit=V  AffineConversion=off
  PS-Simulink Converter3 : nesl_utility_internal/PS-Simulink Converter  PhysicalDomain=network_engine_domain  SubClassName=ps_output  LeftPortType=input  RightPortType=output  PseudoPeriodic=off  Frequencies=[]  VectorFormat=1-D array  Unit=A  AffineConversion=off
  PS-Simulink Converter6 : nesl_utility_internal/PS-Simulink Converter  PhysicalDomain=network_engine_domain  SubClassName=ps_output  LeftPortType=input  RightPortType=output  PseudoPeriodic=off  Frequencies=[]  VectorFormat=1-D array  Unit=MW  AffineConversion=off
  PS-Simulink Converter7 : nesl_utility_internal/PS-Simulink Converter  PhysicalDomain=network_engine_domain  SubClassName=ps_output  LeftPortType=input  RightPortType=output  PseudoPeriodic=off  Frequencies=[]  VectorFormat=1-D array  Unit=MV*A  AffineConversion=off
  Power Sensor (Three-Phase)1 : ee_lib/Sensors & Transducers/Power Sensor (Three-Phase)  load_type=ee.enum.passive.type_balanced.balanced  f0=60 Hz  config=ee.enum.with_neutral.no  rho=1
      settings: InternalSimscapePortConfiguration="{\"Bottom\":[],\"Left\":[{\"id\":\"N1\",\"label\":\"~1\",\"type\":\"foundation.electrical.three_phase\"}],\"Right\":[{\"id\":\"N2\",\"label\":\"~2\",\"type\":\"foundation.electrical.three_phase\"}],\"Top\":[{\"id\":\"Pm\",\"label\":\"P\",\"type\":\"output\"},{\"id\":\"Qm\",\"label\":\"Q\",\"type\":\"output\"}]}"
  a1 : PMIOPort  Side=Left
  ~ : PMIOPort  Port=2  Side=Right
  Out Bus Element : Outport  PortName=mBESS  Element=voltage
  Out Bus Element1 : Outport  PortName=mBESS  Element=current
  Out Bus Element2 : Outport  PortName=mBESS  Element=active power
  Out Bus Element3 : Outport  PortName=mBESS  Element=reactive power
  wires:
  PS-Simulink Converter2/1 -> Out Bus Element/1
  PS-Simulink Converter6/1 -> Low-Pass Filter (Discrete or Continuous)1/1
  PS-Simulink Converter7/1 -> Low-Pass Filter (Discrete or Continuous)/1
  PS-Simulink Converter3/1 -> Out Bus Element1/1
  Low-Pass Filter (Discrete or Continuous)/1 -> Out Bus Element3/1
  Low-Pass Filter (Discrete or Continuous)1/1 -> Out Bus Element2/1
  connections:
  Power Sensor (Three-Phase)1/LConn1 -- Current and Voltage Sensor (Three-Phase)/RConn3
  Current and Voltage Sensor (Three-Phase)/LConn1 -- a1/RConn1
  PS-Simulink Converter2/LConn1 -- Current and Voltage Sensor (Three-Phase)/RConn1
  Current and Voltage Sensor (Three-Phase)/RConn2 -- PS-Simulink Converter3/LConn1
  Power Sensor (Three-Phase)1/LConn2 -- PS-Simulink Converter6/LConn1
  Power Sensor (Three-Phase)1/LConn3 -- PS-Simulink Converter7/LConn1
  ~/RConn1 -- Power Sensor (Three-Phase)1/RConn1

== system IndustrialMicrogrid/MG1 Primary Substation/BESS and Controller/BESS output filter and transformer ==
  10 kvar : ee_lib/Passive/RLC Assemblies/Wye-Connected Load  parameterization=ee.enum.rlc.parameterization.ratedpower  component_structure=ee.enum.rlc.structure.C  component_structure_PQ=ee.enum.rlc.structure.C  R=1 Ohm  L=0.001 H  C=1e-6 F  VRated=microgrid.voltage V  FRated=grid.frequency Hz  P=0 W  Qpos=0 A*V  Qneg=BESS.qBESSFilter A*V  R_parasitic=1e-6 Ohm  G_parasitic=1e-6 1/Ohm  R_parasitic_PQ=1e-6 Ohm  G_parasitic_PQ=1e-6 1/Ohm  Vmag0=microgrid.voltage V  Vang0=0 deg  Freq0=grid.frequency Hz  IL_specify=on  IL_priority=High  IL=[ 0 0 0 ] A  IL_nominal_specify=off  IL_nominal_unit=A  IL_nominal_value=1  VC_specify=on  VC_priority=High  VC=[ 0 0 0 ] V  VC_nominal_specify=off  VC_nominal_unit=V  VC_nominal_value=1
  Electrical Reference1 : fl_lib/Electrical/Electrical Elements/Electrical Reference
  Transformer 1 kV/13.8 kV : Subsystem
      mask Display: image('$imagefile'); % Use "Edit Image" on toolstrip to change.
  "~ " : PMIOPort  Side=Right
  ~ : PMIOPort  Port=2  Side=Left
  connections:
  Electrical Reference1/LConn1 -- 10 kvar/RConn1
  10 kvar/LConn1 -- Transformer 1 kV/13.8 kV/RConn1 -- "~ "/RConn1
  Transformer 1 kV/13.8 kV/LConn1 -- ~/RConn1

== system IndustrialMicrogrid/MG1 Primary Substation/Microgrid Controller/Active and Reactive Power Reference ==
  Bus Element In3 : Inport  PortName=Control Room  Element=PlannedIslandCmd
  Bus Element In6 : Inport  PortName=Control Room  Element=Pref
  Bus Element In1 : Inport  PortName=Control Room  Element=Qref
  Bus Element In5 : Inport  Port=2  PortName=MGController  Element=IslandMGController.MGPlannedIsland.plannedislandP
  Bus Element In4 : Inport  Port=2  PortName=MGController  Element=IslandMGController.MGPlannedIsland.plannedislandQ
  Mux : Mux  Inputs=2
  Saturation : Saturate  UpperLimit=PQUpperLimit  LowerLimit=PQLowerLimit
  Sum : Sum  Inputs=|++
  Sum1 : Sum  Inputs=|++
  Switch : Switch  Criteria=u2 > Threshold  Threshold=0.5  SaturateOnIntegerOverflow=off  InputSameDT=off
  Switch1 : Switch  Criteria=u2 > Threshold  Threshold=0.5  SaturateOnIntegerOverflow=off  InputSameDT=off
  PQref : Outport
  wires:
  Switch/1 -> Mux/1  "Pref"
  Bus Element In5/1 -> Sum/1
  Bus Element In4/1 -> Sum1/1
  Saturation/1 -> PQref/1
  Mux/1 -> Saturation/1  "PQref"
  Bus Element In3/1 -> Switch1/2, Switch/2
  Bus Element In1/1 -> Sum1/2, Switch1/3
  Sum/1 -> Switch/1
  Switch1/1 -> Mux/2  "Qref"
  Bus Element In6/1 -> Sum/2, Switch/3
  Sum1/1 -> Switch1/1

== system IndustrialMicrogrid/MG1 Primary Substation/Microgrid Controller/Black Start ==
  Bus Element In6 : Inport  PortName=Control Room  Element=VFMode1
  Bus Element In1 : Inport  PortName=Control Room  Element=Vref1
  Bus Element In2 : Inport  PortName=Control Room  Element=Fref1
  Bus Element In4 : Inport  PortName=Control Room  Element=BlackStartMG1
  Bus Element In3 : Inport  PortName=Control Room  Element=BlackStartMG1
  Constant : Constant
  If : If
  If Action Subsystem : Subsystem  TreatAsAtomicUnit=on
  If Action Subsystem1 : Subsystem  TreatAsAtomicUnit=on
  Merge : Merge
  Merge1 : Merge
  Switch : Switch  Criteria=u2 > Threshold  Threshold=0.5  SaturateOnIntegerOverflow=off  InputSameDT=off
  Bus Element Out1 : Outport  PortName=BlackStartcontroller1  Element=VFMode1
  Bus Element Out2 : Outport  PortName=BlackStartcontroller1  Element=Vref1
  Bus Element Out3 : Outport  PortName=BlackStartcontroller1  Element=Fref1
  wires:
  Bus Element In6/1 -> Switch/3
  Constant/1 -> Switch/1
  Bus Element In3/1 -> Switch/2
  Switch/1 -> Bus Element Out1/1  "VFMode2"
  Merge/1 -> Bus Element Out2/1  "Vref"
  Merge1/1 -> Bus Element Out3/1  "Fref"
  Bus Element In1/1 -> If Action Subsystem1/1(Control Room)
  If/1 -> If Action Subsystem/Action
  If/2 -> If Action Subsystem1/Action
  If Action Subsystem/1(Out1) -> Merge/1
  If Action Subsystem1/1(Out1) -> Merge/2
  Bus Element In2/1 -> If Action Subsystem1/2(Control Room1)
  If Action Subsystem/2(Out2) -> Merge1/1
  If Action Subsystem1/2(Out2) -> Merge1/2
  Bus Element In4/1 -> If/1
